simulink model "mpc_prueba"  (R2017a)
settings: Solver=ode4  StartTime=0.0  StopTime=0.6  FixedStep=1e-3  RelTol=1e-3
InitFcn:
  | SimulinkInit
values from neighbouring files (symbols this model uses):
  A = [0 1 zeros(1,10) ... (first row only)    [SimulinkInit.m]    (also in TFtoSS.m = [1 2; 3 4]; pruebasstotf.m)
  B = [0 0 ... (first row only)    [SimulinkInit.m]    (also in TFtoSS.m = [1 0; 2 3]; pruebasstotf.m)
  C = [tf1.Numerator{1,1}(3) tf1.Numerator{1,1}(2) tf1.Numerator{1,1}(1) tf1.Numerator{1,2}(3) tf1.Numerator{1,2}(2) tf1.Numerator{1,2}(1) zeros(1,6) ... (first row only)    [SimulinkInit.m]    (also in TFtoSS.m = [1 0; 0 1]; pruebasstotf.m; pruebauGridSF.m = 0.002654)
  D = zeros(2,2)    [SimulinkInit.m]    (also in TFtoSS.m = zeros(2))
libraries: mpclib x1
settings Model: ExtModeTrigMode=oneshot  ExtModeArmWhenConnect=off  Creator=The MathWorks Inc.  LastModifiedBy=carma
settings DataIOCC: SaveFormat=Array  SaveOutput=off  SignalLogging=off  DSMLogging=off  SaveTime=off  SignalLoggingName=sigsOut
settings OptimizationCC: DefaultParameterBehavior=Inlined  UseDivisionForNetSlopeComputation=on  UseFloatMulNetSlope=on  InlineInvariantSignals=on  PassReuseOutputArgsAs=Individual arguments  ExpressionDepthLimit=2147483647  ZeroExternalMemoryAtStartup=off  ZeroInternalMemoryAtStartup=off  NoFixptDivByZeroProtection=on  EfficientFloat2IntCast=on  LifeSpan=1
settings DebuggingCC: SaveWithParameterizedLinksMsg=none  UnderspecifiedInitializationDetection=Classic  MergeDetectMultiDrivingBlocksExec=none  SignalResolutionControl=TryResolveAllWithWarning  MultiTaskDSMMsg=warning  MultiTaskCondExecSysMsg=none  IntegerOverflowMsg=none  ParameterTunabilityLossMsg=error  FcnCallInpInsideContextMsg=warning  StateNameClashWarn=warning  SFUnexpectedBacktrackingDiag=warning  SFNoUnconditionalDefaultTransitionDiag=warning  SFExecutionAtInitializationDiag=none  IntegerSaturationMsg=none
settings HardwareCC: ProdBitPerPointer=32  ProdBitPerSizeT=32  ProdBitPerPtrDiffT=32  ProdLargestAtomicInteger=Long  ProdLargestAtomicFloat=Double  ProdWordSize=32  ProdHWDeviceType=ARM Compatible->ARM Cortex  TargetBitPerPointer=64  TargetBitPerSizeT=64  TargetBitPerPtrDiffT=64  TargetLongLongMode=on  TargetIntDivRoundTo=Zero  TargetEndianess=LittleEndian  TargetWordSize=64  TargetHWDeviceType=MATLAB Host  ProdEqTarget=off
settings ModelReferenceCC: PropagateSignalLabelsOutOfModel=off
settings SFSimCC: MATLABDynamicMemAlloc=off
settings RTWCC: SystemTargetFile=ert.tlc  GenCodeOnly=on  TemplateMakefile=ert_default_tmf  Description=Embedded Coder  GenerateReport=on  IncludeHyperlinkInReport=on  LaunchReport=on  GenerateTraceInfo=on  GenerateTraceReport=on  GenerateTraceReportSl=on  GenerateTraceReportSf=on  GenerateTraceReportEml=on  GenerateCodeMetricsReport=on
settings CodeAppCC: ForceParamTrailComments=on  IgnoreCustomStorageClasses=off  OperatorAnnotations=on  SimulinkDataObjDesc=on  SFDataObjDesc=on  MATLABFcnDesc=on  CustomSymbolStrGlobalVar=rt$N$M  CustomSymbolStrType=$N$M  CustomSymbolStrFcn=$N$M$F  CustomSymbolStrMacro=$N$M  InsertBlockDesc=on  MATLABSourceComments=on
settings ERTTargetCC: GenerateSampleERTMain=on  IncludeMdlTerminateFcn=off  CombineSignalStateStructs=on  SupportAbsoluteTime=off  SupportComplex=off  SupportContinuousTime=on  SupportNonInlinedSFcns=on  InlinedParameterPlacement=NonHierarchical  ERTCustomFileTemplate=example_file_process.tlc  ERTFilePackagingFormat=CompactWithDataFile
settings ConfigComp: CovMetricSettings=dw  CovHtmlReporting=on  CovSaveCumulativeToWorkspaceVar=on  CovSaveSingleToWorkspaceVar=on  CovExternalEMLEnable=off  CovSFcnEnable=off

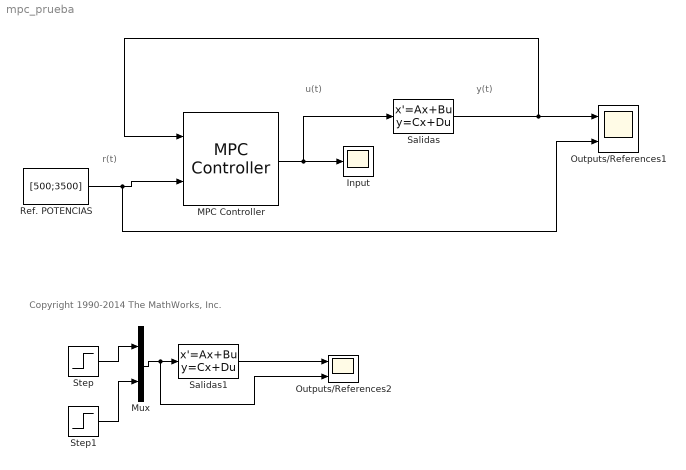
== system mpc_prueba ==
  note: u(t)
  note: y(t)
  note: r(t)
  note: Copyright 1990-2014 The MathWorks, Inc.
  Input : Scope
  MPC Controller : mpclib/MPC Controller  mpcobj=mpcobj  x0=[]  is_multiple=0  enable_value=0  return_u0=off  ref_from_ws=off  ref_signal_name=[]  ref_preview=on  md_from_ws=off  md_signal_name=[]  md_preview=on  from_project=off  project_file=MPCtask.mat  md_inport=off  mv_inport=off  cost_outport=off  return_sequence=off  return_qpstatus=off  return_state=off  state_inport=off  lims_inport=off  ywt_inport=off  is_designfromscratch=0  uwt_inport=off  duwt_inport=off  rhoeps_inport=off  uref_inport=off  n_ts=0.01  n_mv=2  n_md=0  n_ud=0  n_mo=2  n_uo=0  BlockDataType=double  SampleTimeInherited=off  switch_inport=off
  Mux : Mux  Inputs=2
  Outputs/References1 : Scope  NumInputPorts=2
  Outputs/References2 : Scope  NumInputPorts=2
  Ref. POTENCIAS : Constant  Value=[500;3500]
  Salidas : StateSpace  A=A  B=B  C=C  D=D  X0=0
  Salidas1 : StateSpace  A=A  B=B  C=C  D=D  X0=0
  Step : Step  Time=0  After=20  SampleTime=0
  Step1 : Step  Time=0  After=34  SampleTime=0
  wires:
  MPC Controller/1 -> Salidas/1, Input/1
  Salidas/1 -> Outputs/References1/1, MPC Controller/1
  Ref. POTENCIAS/1 -> Outputs/References1/2, MPC Controller/2
  Step/1 -> Mux/1
  Step1/1 -> Mux/2
  Mux/1 -> Outputs/References2/2, Salidas1/1
  Salidas1/1 -> Outputs/References2/1
